simulink model "ejh64a"  (Simulink 3.00)
settings: Solver=ode45  StartTime=0.0  StopTime=15.0  RelTol=1e-3
values from neighbouring files (symbols this model uses):
  K1 = 0.5    [ejh64.m]    (also in ejh65.m)
  K2 = 0.8    [ejh64.m]    (also in ejh65.m)
  x_camino = 0:0.01:10    [ejh64.m]    (also in ejh65.m)
  y_camino = x_camino.^2    [ejh64.m]    (also in ejh65.m)
libraries: simulink_extras x3, dspstat x1
settings Model: OptimizeBlockIOStorage=off  LastModifiedBy=Administrador

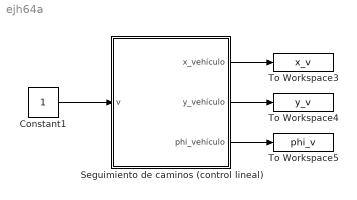
== system ejh64a ==
  Constant1 : Constant  Value=1
  Seguimiento de caminos (control lineal) : Subsystem  mask(Seguimiento de caminos empleando una ley de control lineal){x_inicial=0, y_inicial=0, phi_inicial=0, K1=K1, K2=K2, x_camino=x_camino, y_camino=y_camino}
      mask prompts: x_inicial "Coordenada x inicial del móvil:"; y_inicial "Coordenada y inicial del móvil:"; phi_inicial "Valor inicial de la orientación del móvil:"; K1 "Parámetro K1:"; K2 "Parámetro K2:"; x_camino "Vector con las coordenadas x del camino:"; y_camino "Vector con las coordenadas y del camino:"
      mask help:
      | Este bloque permite simular una estrategia de control lineal para el seguimiento de caminos.
      | A la entrada se dispone de la velocidad del vehículo en cada instante y mediante los parámetros es posible introducir las coordenadas (x,y) del camino. A la salida se obtienen las coordenadas y orientación del vehículo en cada instante.
      mask init:
      | der_x = diff(x_camino);
      | der_y = diff(y_camino);
  To Workspace3 : ToWorkspace  VariableName=x_v  SampleTime=-1  SaveFormat=Matrix
  To Workspace4 : ToWorkspace  VariableName=y_v  SampleTime=-1  SaveFormat=Matrix
  To Workspace5 : ToWorkspace  VariableName=phi_v  SampleTime=-1  SaveFormat=Matrix
  wires:
  Constant1/1 -> Seguimiento de caminos (control lineal)/1(v)
  Seguimiento de caminos (control lineal)/1(x_vehículo) -> To Workspace3/1
  Seguimiento de caminos (control lineal)/3(phi_vehículo) -> To Workspace5/1
  Seguimiento de caminos (control lineal)/2(y_vehículo) -> To Workspace4/1

== system ejh64a/Seguimiento de caminos (control lineal) ==
  v : Inport  Port=1  PortWidth=-1  SampleTime=-1  DataType=auto
      settings: SignalType=auto
  Configuracion síncrona : Subsystem
  Constant : Constant  Value=x_camino
  Constant1 : Constant  Value=y_camino
  Controlador lineal : Subsystem  Orientation=left
  Convertidor : Subsystem  Orientation=left
      mask Description: Este bloque permite transformar la salida del controlador a una señal que será adecuada al vehículo que se desea controlar
  Cálculo de parámetros : Subsystem
  x_vehículo : Outport  Port=1
  y_vehículo : Outport  Port=2
  phi_vehículo : Outport  Port=3
  wires:
  Configuracion síncrona/3(phi_vehículo) -> phi_vehículo/1, Cálculo de parámetros/5(phi_vehiculo)
  Cálculo de parámetros/3(R_c) -> Convertidor/1(R_c)
  v/1 -> Convertidor/3(v), Controlador lineal/2(v), Configuracion síncrona/1(v)
  Configuracion síncrona/2(y_vehículo) -> y_vehículo/1, Cálculo de parámetros/4(y_vehiculo)
  Configuracion síncrona/1(x_vehículo) -> x_vehículo/1, Cálculo de parámetros/3(x_vehiculo)
  Convertidor/1(w) -> Configuracion síncrona/2(w)
  Cálculo de parámetros/1(epsilon) -> Controlador lineal/3(epsilon)
  Controlador lineal/1(u_cont) -> Convertidor/4(u_cont)
  Cálculo de parámetros/2(fi_gorro) -> Convertidor/2(fi_gorro), Controlador lineal/1(fi_gorro)
  Constant1/1 -> Cálculo de parámetros/2(y_camino)
  Constant/1 -> Cálculo de parámetros/1(x_camino)

== system ejh64a/Seguimiento de caminos (control lineal)/Configuracion síncrona ==
  v : Inport  Port=1  PortWidth=-1  SampleTime=-1  DataType=auto
      settings: SignalType=auto
  w : Inport  Port=2  PortWidth=-1  SampleTime=-1  DataType=auto
      settings: SignalType=auto
  Fcn : Fcn  Expr=-sin(u)
  Fcn1 : Fcn  Expr=cos(u)
  Integrator : Integrator  ExternalReset=none  InitialConditionSource=internal  InitialCondition=phi_inicial  LimitOutput=off  UpperSaturationLimit=inf  LowerSaturationLimit=-inf  ShowSaturationPort=off  ShowStatePort=off  AbsoluteTolerance=auto
  Integrator1 : Integrator  ExternalReset=none  InitialConditionSource=internal  InitialCondition=x_inicial  LimitOutput=off  UpperSaturationLimit=inf  LowerSaturationLimit=-inf  ShowSaturationPort=off  ShowStatePort=off  AbsoluteTolerance=auto
  Integrator2 : Integrator  ExternalReset=none  InitialConditionSource=internal  InitialCondition=y_inicial  LimitOutput=off  UpperSaturationLimit=inf  LowerSaturationLimit=-inf  ShowSaturationPort=off  ShowStatePort=off  AbsoluteTolerance=auto
  Product : Product  Inputs=2  SaturateOnIntegerOverflow=on
  Product1 : Product  Inputs=2  SaturateOnIntegerOverflow=on
  x_vehículo : Outport  Port=1
  y_vehículo : Outport  Port=2
  phi_vehículo : Outport  Port=3
  wires:
  Fcn1/1 -> Product1/2
  w/1 -> Integrator/1
  v/1 -> Product1/1, Product/1
  Integrator2/1 -> y_vehículo/1
  Integrator1/1 -> x_vehículo/1
  Integrator/1 -> phi_vehículo/1, Fcn1/1, Fcn/1
  Fcn/1 -> Product/2
  Product/1 -> Integrator1/1
  Product1/1 -> Integrator2/1

== system ejh64a/Seguimiento de caminos (control lineal)/Controlador lineal ==
  fi_gorro : Inport  Port=1  PortWidth=-1  SampleTime=-1  DataType=auto
      settings: SignalType=auto
  v : Inport  Port=2  PortWidth=-1  SampleTime=-1  DataType=auto
      settings: SignalType=auto
  epsilon : Inport  Port=3  PortWidth=-1  SampleTime=-1  DataType=auto
      settings: SignalType=auto
  Abs : Abs
  Gain : Gain  Gain=K1  SaturateOnIntegerOverflow=on
  Gain1 : Gain  Gain=K2  SaturateOnIntegerOverflow=on
  Product : Product  Inputs=2  SaturateOnIntegerOverflow=on
  Product1 : Product  Inputs=2  SaturateOnIntegerOverflow=on
  Sum : Sum  Inputs=--  SaturateOnIntegerOverflow=on
  u_cont : Outport  Port=1  InitialOutput=0
  wires:
  Gain/1 -> Product/1
  v/1 -> Product/2, Abs/1
  Gain1/1 -> Product1/1
  Abs/1 -> Product1/2
  Product/1 -> Sum/1
  Product1/1 -> Sum/2
  epsilon/1 -> Gain/1
  Sum/1 -> u_cont/1
  fi_gorro/1 -> Gain1/1

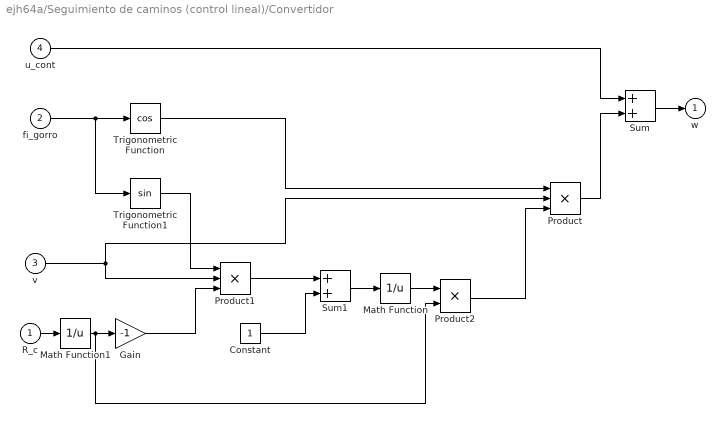
== system ejh64a/Seguimiento de caminos (control lineal)/Convertidor ==
  R_c : Inport  Port=1  PortWidth=-1  SampleTime=-1  DataType=auto
      settings: SignalType=auto
  fi_gorro : Inport  Port=2  PortWidth=-1  SampleTime=-1  DataType=auto
      settings: SignalType=auto
  v : Inport  Port=3  PortWidth=-1  SampleTime=-1  DataType=auto
      settings: SignalType=auto
  u_cont : Inport  Port=4  PortWidth=-1  SampleTime=-1  DataType=auto
      settings: SignalType=auto
  Constant : Constant  Value=1
  Gain : Gain  Gain=-1  SaturateOnIntegerOverflow=on
  Math Function : Math  Operator=reciprocal  OutputSignalType=auto
  Math Function1 : Math  Operator=reciprocal  OutputSignalType=auto
  Product : Product  Inputs=3  SaturateOnIntegerOverflow=on
  Product1 : Product  Inputs=3  SaturateOnIntegerOverflow=on
  Product2 : Product  Inputs=2  SaturateOnIntegerOverflow=on
  Sum : Sum  Inputs=++  SaturateOnIntegerOverflow=on
  Sum1 : Sum  Inputs=++  SaturateOnIntegerOverflow=on
  Trigonometric Function : Trigonometry  Operator=cos  OutputSignalType=auto
  Trigonometric Function1 : Trigonometry  Operator=sin  OutputSignalType=auto
  w : Outport  Port=1  InitialOutput=0
  wires:
  Math Function1/1 -> Gain/1, Product2/2
  R_c/1 -> Math Function1/1
  fi_gorro/1 -> Trigonometric Function/1, Trigonometric Function1/1
  Trigonometric Function1/1 -> Product1/1
  Gain/1 -> Product1/3
  Product1/1 -> Sum1/1
  Constant/1 -> Sum1/2
  Sum1/1 -> Math Function/1
  Trigonometric Function/1 -> Product/1
  v/1 -> Product1/2, Product/2
  Math Function/1 -> Product2/1
  Product/1 -> Sum/2
  u_cont/1 -> Sum/1
  Sum/1 -> w/1
  Product2/1 -> Product/3

== system ejh64a/Seguimiento de caminos (control lineal)/Cálculo de parámetros ==
  x_camino : Inport  Port=1  PortWidth=-1  SampleTime=-1  DataType=auto
      settings: SignalType=auto
  y_camino : Inport  Port=2  PortWidth=-1  SampleTime=-1  DataType=auto
      settings: SignalType=auto
  x_vehiculo : Inport  Port=3  PortWidth=-1  SampleTime=-1  DataType=auto
      settings: SignalType=auto
  y_vehiculo : Inport  Port=4  PortWidth=-1  SampleTime=-1  DataType=auto
      settings: SignalType=auto
  phi_vehiculo : Inport  Port=5  PortWidth=-1  SampleTime=-1  DataType=auto
      settings: SignalType=auto
  Cálculo de phi gorro : Subsystem
  Degrees to Radians : simulink_extras/Transformations/Degrees to Radians
  Subsystem : Subsystem
  epsilon : Outport  Port=1
  fi_gorro : Outport  Port=2
  R_c : Outport  Port=3
  wires:
  x_camino/1 -> Subsystem/1(x_camino)
  y_camino/1 -> Subsystem/2(y_camino)
  y_vehiculo/1 -> Subsystem/4(y_vehiculo)
  x_vehiculo/1 -> Subsystem/3(x_vehiculo)
  Subsystem/3(R_c) -> R_c/1
  phi_vehiculo/1 -> Cálculo de phi gorro/1(fi_vehiculo)
  Degrees to Radians/1 -> fi_gorro/1
  Cálculo de phi gorro/1(fi_go_mo) -> Degrees to Radians/1
  Subsystem/1(distancia) -> epsilon/1
  Subsystem/2(indice) -> Cálculo de phi gorro/2(indice)

== system ejh64a/Seguimiento de caminos (control lineal)/Cálculo de parámetros/Cálculo de phi gorro ==
  fi_vehiculo : Inport  Port=1  PortWidth=-1  SampleTime=-1  DataType=auto
      settings: SignalType=auto
  indice : Inport  Port=2  PortWidth=-1  SampleTime=-1  DataType=auto
      settings: SignalType=auto
  Subsystem : Subsystem
      mask Type: Pasa phi a un ángulo entre -180 y 180
      mask Description: Pasa phi a un ángulo entre -180 y 180
      mask Help: Pasa phi a un ángulo entre -180 y 180
  Subsystem1 : Subsystem
  Subsystem2 : Subsystem
      mask Description: Pasa phi gorro al intervalo -180,180
  suma : Sum  Inputs=+-  SaturateOnIntegerOverflow=on
  fi_go_mo : Outport  Port=1
  wires:
  Subsystem2/1(fi_go_mo) -> fi_go_mo/1
  suma/1 -> Subsystem2/1(fi_gorro)
  Subsystem/1(fi_veh_mod) -> suma/1
  indice/1 -> Subsystem1/1(indice)
  fi_vehiculo/1 -> Subsystem/1(fi_vehiculo)
  Subsystem1/1(fi_camino) -> suma/2

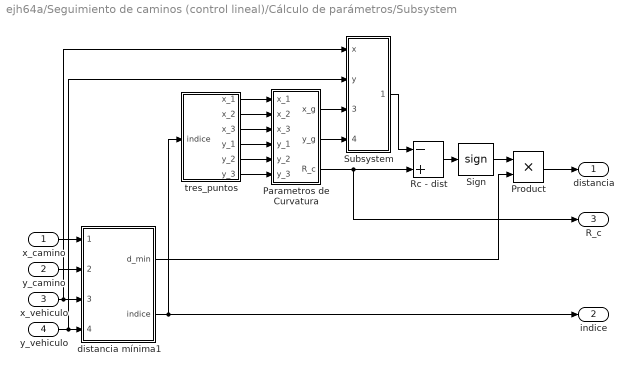
== system ejh64a/Seguimiento de caminos (control lineal)/Cálculo de parámetros/Subsystem ==
  x_camino : Inport  Port=1  PortWidth=-1  SampleTime=-1  DataType=auto
      settings: SignalType=auto
  y_camino : Inport  Port=2  PortWidth=-1  SampleTime=-1  DataType=auto
      settings: SignalType=auto
  x_vehiculo : Inport  Port=3  PortWidth=-1  SampleTime=-1  DataType=auto
      settings: SignalType=auto
  y_vehiculo : Inport  Port=4  PortWidth=-1  SampleTime=-1  DataType=auto
      settings: SignalType=auto
  Parametros de Curvatura : Subsystem
  Product : Product  Inputs=2  SaturateOnIntegerOverflow=on
  Rc - dist : Sum  Inputs=-+  SaturateOnIntegerOverflow=on
  Sign : Signum
  Subsystem : Subsystem
  distancia mínima1 : Subsystem
  tres_puntos : Subsystem
  distancia : Outport  Port=1
  indice : Outport  Port=2
  R_c : Outport  Port=3
  wires:
  distancia mínima1/2(indice) -> tres_puntos/1(indice), indice/1
  Parametros de Curvatura/3(R_c) -> R_c/1, Rc - dist/2
  y_vehiculo/1 -> Subsystem/2(y), distancia mínima1/4(y_vehiculo)
  x_vehiculo/1 -> Subsystem/1(x), distancia mínima1/3(x_vehiculo)
  tres_puntos/4(y_1) -> Parametros de Curvatura/4(y_1)
  tres_puntos/1(x_1) -> Parametros de Curvatura/1(x_1)
  Product/1 -> distancia/1
  y_camino/1 -> distancia mínima1/2(y_camino)
  x_camino/1 -> distancia mínima1/1(x_camino)
  tres_puntos/6(y_3) -> Parametros de Curvatura/6(y_3)
  tres_puntos/5(y_2) -> Parametros de Curvatura/5(y_2)
  tres_puntos/3(x_3) -> Parametros de Curvatura/3(x_3)
  tres_puntos/2(x_2) -> Parametros de Curvatura/2(x_2)
  distancia mínima1/1(d_min) -> Product/2
  Sign/1 -> Product/1
  Parametros de Curvatura/1(x_g) -> Subsystem/3(x_g)
  Parametros de Curvatura/2(y_g) -> Subsystem/4(y_g)
  Subsystem/1(dist) -> Rc - dist/1
  Rc - dist/1 -> Sign/1

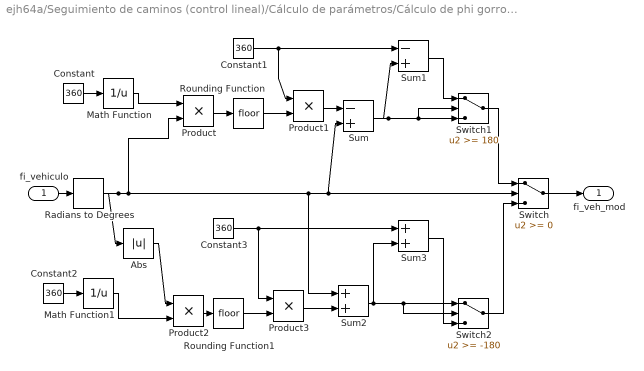
== system ejh64a/Seguimiento de caminos (control lineal)/Cálculo de parámetros/Cálculo de phi gorro/Subsystem ==
  fi_vehiculo : Inport  Port=1  PortWidth=-1  SampleTime=-1  DataType=auto
      settings: SignalType=auto
  Abs : Abs
  Constant{,1..3} (4 alike) : Constant  Value=360
  Math Function : Math  Operator=reciprocal  OutputSignalType=auto
  Math Function1 : Math  Operator=reciprocal  OutputSignalType=auto
  Product{,1..3} (4 alike) : Product  Inputs=2  SaturateOnIntegerOverflow=on
  Radians to Degrees : simulink_extras/Transformations/Radians to Degrees
  Rounding Function : Rounding  Operator=floor
  Rounding Function1 : Rounding  Operator=floor
  Sum : Sum  Inputs=-+  SaturateOnIntegerOverflow=on
  Sum1 : Sum  Inputs=-+  SaturateOnIntegerOverflow=on
  Sum2 : Sum  Inputs=++  SaturateOnIntegerOverflow=on
  Sum3 : Sum  Inputs=++  SaturateOnIntegerOverflow=on
  Switch : Switch  Threshold=0
  Switch1 : Switch  Threshold=180
  Switch2 : Switch  Threshold=-180
  fi_veh_mod : Outport  Port=1
  wires:
  Radians to Degrees/1 -> Abs/1, Sum2/1, Sum/2, Switch/2, Product/2
  fi_vehiculo/1 -> Radians to Degrees/1
  Abs/1 -> Product2/1
  Sum2/1 -> Switch2/2, Switch2/1, Sum3/2
  Sum3/1 -> Switch2/3
  Product2/1 -> Rounding Function1/1
  Math Function1/1 -> Product2/2
  Constant2/1 -> Math Function1/1
  Product3/1 -> Sum2/2
  Rounding Function1/1 -> Product3/2
  Switch2/1 -> Switch/3
  Constant3/1 -> Sum3/1, Product3/1
  Sum1/1 -> Switch1/1
  Sum/1 -> Switch1/2, Switch1/3, Sum1/2
  Constant1/1 -> Sum1/1, Product1/1
  Product1/1 -> Sum/1
  Rounding Function/1 -> Product1/2
  Product/1 -> Rounding Function/1
  Constant/1 -> Math Function/1
  Math Function/1 -> Product/1
  Switch1/1 -> Switch/1
  Switch/1 -> fi_veh_mod/1

== system ejh64a/Seguimiento de caminos (control lineal)/Cálculo de parámetros/Cálculo de phi gorro/Subsystem1 ==
  indice : Inport  Port=1  PortWidth=-1  SampleTime=-1  DataType=auto
      settings: SignalType=auto
  Constant : Constant  Value=90
  Constant1 : Constant  Value=360
  Look-Up Table : Lookup  InputValues=1:length(der_x)  OutputValues=der_x(1:length(der_x))
  Look-Up Table1 : Lookup  InputValues=1:length(der_y)  OutputValues=der_y(1:length(der_y))
  Radians to Degrees : simulink_extras/Transformations/Radians to Degrees
  Sum : Sum  Inputs=+-  SaturateOnIntegerOverflow=on
  Sum1 : Sum  Inputs=++  SaturateOnIntegerOverflow=on
  Switch : Switch  Threshold=-180
  Trigonometric Function : Trigonometry  Operator=atan2  OutputSignalType=auto
  fi_camino : Outport  Port=1
  wires:
  indice/1 -> Look-Up Table/1, Look-Up Table1/1
  Switch/1 -> fi_camino/1
  Sum1/1 -> Switch/3
  Sum/1 -> Switch/2, Sum1/1, Switch/1
  Constant1/1 -> Sum1/2
  Constant/1 -> Sum/2
  Radians to Degrees/1 -> Sum/1
  Trigonometric Function/1 -> Radians to Degrees/1
  Look-Up Table/1 -> Trigonometric Function/2
  Look-Up Table1/1 -> Trigonometric Function/1

== system ejh64a/Seguimiento de caminos (control lineal)/Cálculo de parámetros/Cálculo de phi gorro/Subsystem2 ==
  fi_gorro : Inport  Port=1  PortWidth=-1  SampleTime=-1  DataType=auto
      settings: SignalType=auto
  Constant1 : Constant  Value=360
  Constant2 : Constant  Value=360
  Sum1 : Sum  Inputs=-+  SaturateOnIntegerOverflow=on
  Sum2 : Sum  Inputs=++  SaturateOnIntegerOverflow=on
  Switch : Switch  Threshold=180
  Switch1 : Switch  Threshold=0
  Switch2 : Switch  Threshold=-180
  fi_go_mo : Outport  Port=1
  wires:
  Constant2/1 -> Sum2/2
  fi_gorro/1 -> Sum2/1, Switch2/2, Switch2/1, Switch/2, Switch/3, Switch1/2, Sum1/2
  Sum2/1 -> Switch2/3
  Sum1/1 -> Switch/1
  Constant1/1 -> Sum1/1
  Switch2/1 -> Switch1/3
  Switch/1 -> Switch1/1
  Switch1/1 -> fi_go_mo/1

== system ejh64a/Seguimiento de caminos (control lineal)/Cálculo de parámetros/Subsystem/Parametros de Curvatura ==
  x_1 : Inport  Port=1  PortWidth=-1  SampleTime=-1  DataType=auto
      settings: SignalType=auto
  x_2 : Inport  Port=2  PortWidth=-1  SampleTime=-1  DataType=auto
      settings: SignalType=auto
  x_3 : Inport  Port=3  PortWidth=-1  SampleTime=-1  DataType=auto
      settings: SignalType=auto
  y_1 : Inport  Port=4  PortWidth=-1  SampleTime=-1  DataType=auto
      settings: SignalType=auto
  y_2 : Inport  Port=5  PortWidth=-1  SampleTime=-1  DataType=auto
      settings: SignalType=auto
  y_3 : Inport  Port=6  PortWidth=-1  SampleTime=-1  DataType=auto
      settings: SignalType=auto
  Radio de  Curvatura : Subsystem
  coordenada x c. curvatura : Subsystem
  coordenada y c. curvatura : Subsystem
  x_g : Outport  Port=1  InitialOutput=0
  y_g : Outport  Port=2  InitialOutput=0
  R_c : Outport  Port=3  InitialOutput=0
  wires:
  y_3/1 -> coordenada x c. curvatura/6(y_3), coordenada y c. curvatura/6(y_3)
  y_2/1 -> coordenada y c. curvatura/5(y_2), coordenada x c. curvatura/5(y_2)
  y_1/1 -> Radio de  Curvatura/4(y_1), coordenada x c. curvatura/4(y_1), coordenada y c. curvatura/4(y_1)
  x_3/1 -> coordenada y c. curvatura/3(x_3), coordenada x c. curvatura/3(x_3)
  x_2/1 -> coordenada y c. curvatura/2(x_2), coordenada x c. curvatura/2(x_2)
  x_1/1 -> Radio de  Curvatura/2(x_1), coordenada y c. curvatura/1(x_1), coordenada x c. curvatura/1(x_1)
  coordenada x c. curvatura/1(x_g) -> Radio de  Curvatura/1(x_g), x_g/1
  coordenada y c. curvatura/1(y_g) -> Radio de  Curvatura/3(y_g), y_g/1
  Radio de  Curvatura/1(R_c) -> R_c/1

== system ejh64a/Seguimiento de caminos (control lineal)/Cálculo de parámetros/Subsystem/Subsystem ==
  x : Inport  Port=1  PortWidth=-1  SampleTime=-1  DataType=auto
      settings: SignalType=auto
  y : Inport  Port=2  PortWidth=-1  SampleTime=-1  DataType=auto
      settings: SignalType=auto
  x_g : Inport  Port=3  PortWidth=-1  SampleTime=-1  DataType=auto
      settings: SignalType=auto
  y_g : Inport  Port=4  PortWidth=-1  SampleTime=-1  DataType=auto
      settings: SignalType=auto
  Math Function2 : Math  Operator=sqrt  OutputSignalType=auto
  Math Function3 : Math  Operator=square  OutputSignalType=auto
  Math Function4 : Math  Operator=square  OutputSignalType=auto
  Sum : Sum  Inputs=+-  SaturateOnIntegerOverflow=on
  Sum1 : Sum  Inputs=+-  SaturateOnIntegerOverflow=on
  Sum2 : Sum  Inputs=++  SaturateOnIntegerOverflow=on
  dist : Outport  Port=1  InitialOutput=0
  wires:
  Sum2/1 -> Math Function2/1
  Math Function4/1 -> Sum2/2
  Sum1/1 -> Math Function4/1
  Math Function3/1 -> Sum2/1
  Sum/1 -> Math Function3/1
  y/1 -> Sum1/1
  x_g/1 -> Sum/2
  x/1 -> Sum/1
  y_g/1 -> Sum1/2
  Math Function2/1 -> dist/1

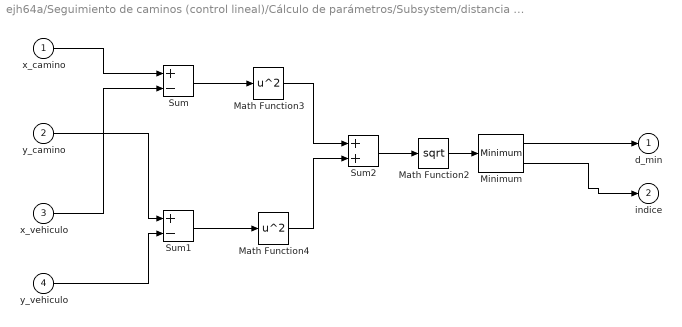
== system ejh64a/Seguimiento de caminos (control lineal)/Cálculo de parámetros/Subsystem/distancia mínima1 ==
  x_camino : Inport  Port=1  PortWidth=-1  SampleTime=-1  DataType=auto
      settings: SignalType=auto
  y_camino : Inport  Port=2  PortWidth=-1  SampleTime=-1  DataType=auto
      settings: SignalType=auto
  x_vehiculo : Inport  Port=3  PortWidth=-1  SampleTime=-1  DataType=auto
      settings: SignalType=auto
  y_vehiculo : Inport  Port=4  PortWidth=-1  SampleTime=-1  DataType=auto
      settings: SignalType=auto
  Math Function2 : Math  Operator=sqrt  OutputSignalType=auto
  Math Function3 : Math  Operator=square  OutputSignalType=auto
  Math Function4 : Math  Operator=square  OutputSignalType=auto
  Minimum : dspstat/Minimum
  Sum : Sum  Inputs=+-  SaturateOnIntegerOverflow=on
  Sum1 : Sum  Inputs=+-  SaturateOnIntegerOverflow=on
  Sum2 : Sum  Inputs=++  SaturateOnIntegerOverflow=on
  d_min : Outport  Port=1  InitialOutput=0
  indice : Outport  Port=2  InitialOutput=0
  wires:
  Minimum/2 -> indice/1
  Minimum/1 -> d_min/1
  Math Function2/1 -> Minimum/1
  Sum2/1 -> Math Function2/1
  Math Function4/1 -> Sum2/2
  Sum1/1 -> Math Function4/1
  Math Function3/1 -> Sum2/1
  Sum/1 -> Math Function3/1
  y_vehiculo/1 -> Sum1/2
  y_camino/1 -> Sum1/1
  x_vehiculo/1 -> Sum/2
  x_camino/1 -> Sum/1

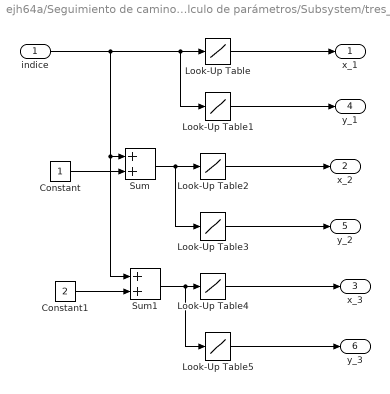
== system ejh64a/Seguimiento de caminos (control lineal)/Cálculo de parámetros/Subsystem/tres_puntos ==
  indice : Inport  Port=1  PortWidth=-1  SampleTime=-1  DataType=auto
      settings: SignalType=auto
  Constant : Constant  Value=1
  Constant1 : Constant  Value=2
  Look-Up Table : Lookup  InputValues=1:length(x_camino)  OutputValues=x_camino(1:length(x_camino))
  Look-Up Table1 : Lookup  InputValues=1:length(y_camino)  OutputValues=y_camino(1:length(y_camino))
  Look-Up Table2 : Lookup  InputValues=1:length(x_camino)  OutputValues=x_camino(1:length(x_camino))
  Look-Up Table3 : Lookup  InputValues=1:length(y_camino)  OutputValues=y_camino(1:length(y_camino))
  Look-Up Table4 : Lookup  InputValues=1:length(x_camino)  OutputValues=x_camino(1:length(x_camino))
  Look-Up Table5 : Lookup  InputValues=1:length(y_camino)  OutputValues=y_camino(1:length(y_camino))
  Sum : Sum  Inputs=++  SaturateOnIntegerOverflow=on
  Sum1 : Sum  Inputs=++  SaturateOnIntegerOverflow=on
  x_1 : Outport  Port=1
  x_2 : Outport  Port=2
  x_3 : Outport  Port=3
  y_1 : Outport  Port=4
  y_2 : Outport  Port=5
  y_3 : Outport  Port=6
  wires:
  Sum1/1 -> Look-Up Table5/1, Look-Up Table4/1
  Look-Up Table4/1 -> x_3/1
  Look-Up Table5/1 -> y_3/1
  Constant1/1 -> Sum1/2
  Look-Up Table1/1 -> y_1/1
  Sum/1 -> Look-Up Table3/1, Look-Up Table2/1
  Look-Up Table3/1 -> y_2/1
  Look-Up Table2/1 -> x_2/1
  Constant/1 -> Sum/2
  indice/1 -> Sum1/1, Sum/1, Look-Up Table1/1, Look-Up Table/1
  Look-Up Table/1 -> x_1/1

== system ejh64a/Seguimiento de caminos (control lineal)/Cálculo de parámetros/Subsystem/Parametros de Curvatura/Radio de  Curvatura ==
  x_g : Inport  Port=1  PortWidth=-1  SampleTime=-1  DataType=auto
      settings: SignalType=auto
  x_1 : Inport  Port=2  PortWidth=-1  SampleTime=-1  DataType=auto
      settings: SignalType=auto
  y_g : Inport  Port=3  PortWidth=-1  SampleTime=-1  DataType=auto
      settings: SignalType=auto
  y_1 : Inport  Port=4  PortWidth=-1  SampleTime=-1  DataType=auto
      settings: SignalType=auto
  Math Function : Math  Operator=square  OutputSignalType=auto
  Math Function1 : Math  Operator=sqrt  OutputSignalType=auto
  Math Function2 : Math  Operator=square  OutputSignalType=auto
  Sum : Sum  Inputs=+-  SaturateOnIntegerOverflow=on
  Sum1 : Sum  Inputs=+-  SaturateOnIntegerOverflow=on
  Sum2 : Sum  Inputs=++  SaturateOnIntegerOverflow=on
  R_c : Outport  Port=1  InitialOutput=0
  wires:
  Math Function1/1 -> R_c/1
  Sum2/1 -> Math Function1/1
  Math Function2/1 -> Sum2/2
  Math Function/1 -> Sum2/1
  Sum1/1 -> Math Function2/1
  Sum/1 -> Math Function/1
  y_g/1 -> Sum1/2
  y_1/1 -> Sum1/1
  x_1/1 -> Sum/1
  x_g/1 -> Sum/2

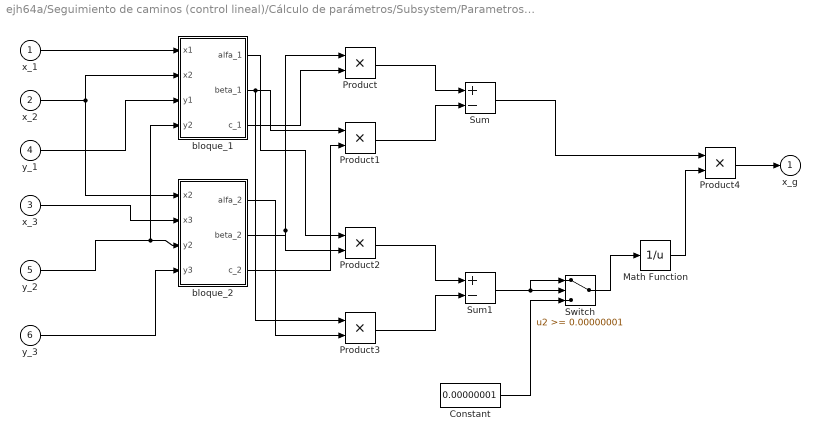
== system ejh64a/Seguimiento de caminos (control lineal)/Cálculo de parámetros/Subsystem/Parametros de Curvatura/coordenada x c. curvatura ==
  x_1 : Inport  Port=1  PortWidth=-1  SampleTime=-1  DataType=auto
      settings: SignalType=auto
  x_2 : Inport  Port=2  PortWidth=-1  SampleTime=-1  DataType=auto
      settings: SignalType=auto
  x_3 : Inport  Port=3  PortWidth=-1  SampleTime=-1  DataType=auto
      settings: SignalType=auto
  y_1 : Inport  Port=4  PortWidth=-1  SampleTime=-1  DataType=auto
      settings: SignalType=auto
  y_2 : Inport  Port=5  PortWidth=-1  SampleTime=-1  DataType=auto
      settings: SignalType=auto
  y_3 : Inport  Port=6  PortWidth=-1  SampleTime=-1  DataType=auto
      settings: SignalType=auto
  Constant : Constant  Value=0.00000001
  Math Function : Math  Operator=reciprocal  OutputSignalType=auto
  Product{,1..4} (5 alike) : Product  Inputs=2  SaturateOnIntegerOverflow=on
  Sum : Sum  Inputs=+-  SaturateOnIntegerOverflow=on
  Sum1 : Sum  Inputs=+-  SaturateOnIntegerOverflow=on
  Switch : Switch  Threshold=0.00000001
  bloque_1 : Subsystem
  bloque_2 : Subsystem
  x_g : Outport  Port=1  InitialOutput=0
  wires:
  Switch/1 -> Math Function/1
  Constant/1 -> Switch/3
  Sum1/1 -> Switch/1, Switch/2
  Product4/1 -> x_g/1
  Product/1 -> Sum/1
  Product1/1 -> Sum/2
  Product2/1 -> Sum1/1
  Product3/1 -> Sum1/2
  Math Function/1 -> Product4/2
  bloque_1/3(c_1) -> Product/2
  bloque_2/3(c_2) -> Product1/2
  bloque_2/2(beta_2) -> Product/1, Product2/2
  bloque_1/1(alfa_1) -> Product2/1
  bloque_1/2(beta_1) -> Product1/1, Product3/1
  bloque_2/1(alfa_2) -> Product3/2
  x_1/1 -> bloque_1/1(x1)
  x_2/1 -> bloque_1/2(x2), bloque_2/1(x2)
  y_1/1 -> bloque_1/3(y1)
  x_3/1 -> bloque_2/2(x3)
  y_2/1 -> bloque_2/3(y2), bloque_1/4(y2)
  y_3/1 -> bloque_2/4(y3)
  Sum/1 -> Product4/1

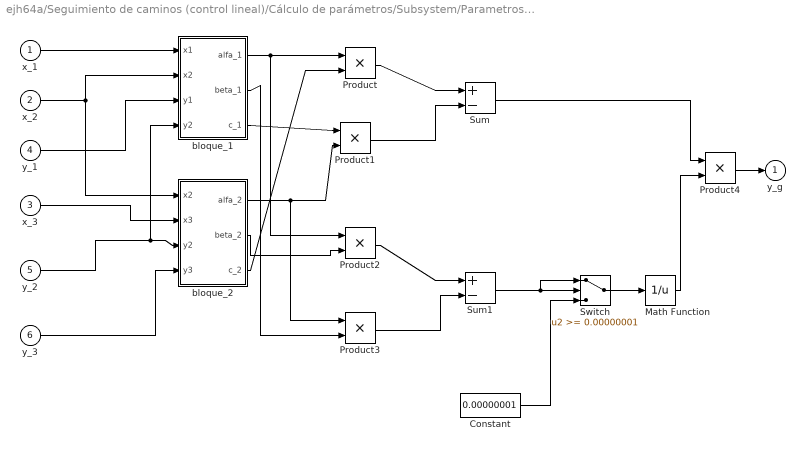
== system ejh64a/Seguimiento de caminos (control lineal)/Cálculo de parámetros/Subsystem/Parametros de Curvatura/coordenada y c. curvatura ==
  x_1 : Inport  Port=1  PortWidth=-1  SampleTime=-1  DataType=auto
      settings: SignalType=auto
  x_2 : Inport  Port=2  PortWidth=-1  SampleTime=-1  DataType=auto
      settings: SignalType=auto
  x_3 : Inport  Port=3  PortWidth=-1  SampleTime=-1  DataType=auto
      settings: SignalType=auto
  y_1 : Inport  Port=4  PortWidth=-1  SampleTime=-1  DataType=auto
      settings: SignalType=auto
  y_2 : Inport  Port=5  PortWidth=-1  SampleTime=-1  DataType=auto
      settings: SignalType=auto
  y_3 : Inport  Port=6  PortWidth=-1  SampleTime=-1  DataType=auto
      settings: SignalType=auto
  Constant : Constant  Value=0.00000001
  Math Function : Math  Operator=reciprocal  OutputSignalType=auto
  Product{,1..4} (5 alike) : Product  Inputs=2  SaturateOnIntegerOverflow=on
  Sum : Sum  Inputs=+-  SaturateOnIntegerOverflow=on
  Sum1 : Sum  Inputs=+-  SaturateOnIntegerOverflow=on
  Switch : Switch  Threshold=0.00000001
  bloque_1 : Subsystem
  bloque_2 : Subsystem
  y_g : Outport  Port=1  InitialOutput=0
  wires:
  Constant/1 -> Switch/3
  Sum1/1 -> Switch/1, Switch/2
  Switch/1 -> Math Function/1
  Math Function/1 -> Product4/2
  Product4/1 -> y_g/1
  bloque_2/3(c_2) -> Product/2
  bloque_1/3(c_1) -> Product1/1
  bloque_1/1(alfa_1) -> Product/1, Product2/1
  bloque_2/2(beta_2) -> Product2/2
  bloque_1/2(beta_1) -> Product3/2
  bloque_2/1(alfa_2) -> Product1/2, Product3/1
  Product/1 -> Sum/1
  Product1/1 -> Sum/2
  Product2/1 -> Sum1/1
  Product3/1 -> Sum1/2
  x_1/1 -> bloque_1/1(x1)
  x_2/1 -> bloque_1/2(x2), bloque_2/1(x2)
  y_1/1 -> bloque_1/3(y1)
  x_3/1 -> bloque_2/2(x3)
  y_2/1 -> bloque_2/3(y2), bloque_1/4(y2)
  y_3/1 -> bloque_2/4(y3)
  Sum/1 -> Product4/1

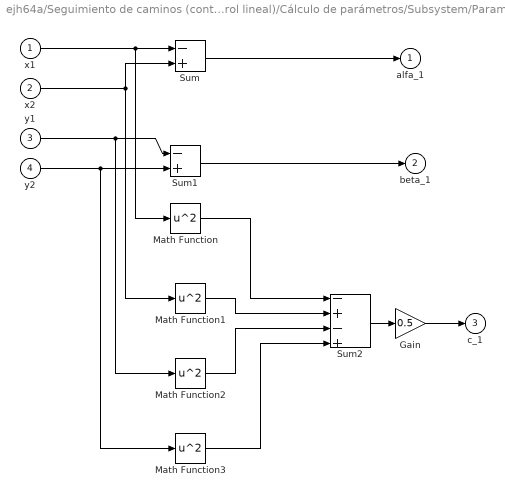
== system ejh64a/Seguimiento de caminos (control lineal)/Cálculo de parámetros/Subsystem/Parametros de Curvatura/coordenada x c. curvatura/bloque_1 ==
  x1 : Inport  Port=1  PortWidth=-1  SampleTime=-1  DataType=auto
      settings: SignalType=auto
  x2 : Inport  Port=2  PortWidth=-1  SampleTime=-1  DataType=auto
      settings: SignalType=auto
  y1 : Inport  Port=3  PortWidth=-1  SampleTime=-1  DataType=auto
      settings: SignalType=auto
  y2 : Inport  Port=4  PortWidth=-1  SampleTime=-1  DataType=auto
      settings: SignalType=auto
  Gain : Gain  Gain=0.5  SaturateOnIntegerOverflow=on
  Math Function{,1..3} (4 alike) : Math  Operator=square  OutputSignalType=auto
  Sum : Sum  Inputs=-+  SaturateOnIntegerOverflow=on
  Sum1 : Sum  Inputs=-+  SaturateOnIntegerOverflow=on
  Sum2 : Sum  Inputs=-+-+  SaturateOnIntegerOverflow=on
  alfa_1 : Outport  Port=1  InitialOutput=0
  beta_1 : Outport  Port=2  InitialOutput=0
  c_1 : Outport  Port=3  InitialOutput=0
  wires:
  Sum/1 -> alfa_1/1
  Sum1/1 -> beta_1/1
  x1/1 -> Sum/1, Math Function/1
  x2/1 -> Sum/2, Math Function1/1
  y1/1 -> Sum1/1, Math Function2/1
  y2/1 -> Sum1/2, Math Function3/1
  Math Function/1 -> Sum2/1
  Math Function1/1 -> Sum2/2
  Math Function2/1 -> Sum2/3
  Math Function3/1 -> Sum2/4
  Sum2/1 -> Gain/1
  Gain/1 -> c_1/1

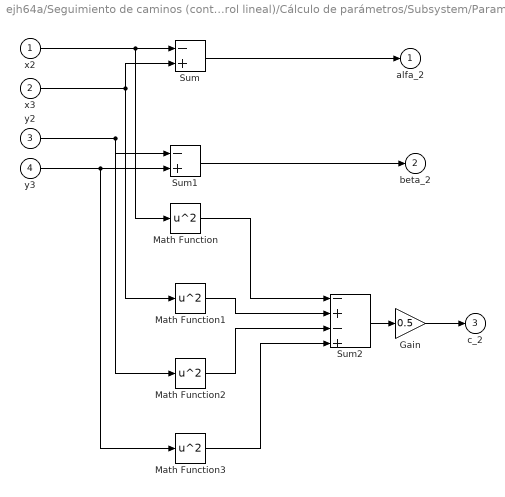
== system ejh64a/Seguimiento de caminos (control lineal)/Cálculo de parámetros/Subsystem/Parametros de Curvatura/coordenada x c. curvatura/bloque_2 ==
  x2 : Inport  Port=1  PortWidth=-1  SampleTime=-1  DataType=auto
      settings: SignalType=auto
  x3 : Inport  Port=2  PortWidth=-1  SampleTime=-1  DataType=auto
      settings: SignalType=auto
  y2 : Inport  Port=3  PortWidth=-1  SampleTime=-1  DataType=auto
      settings: SignalType=auto
  y3 : Inport  Port=4  PortWidth=-1  SampleTime=-1  DataType=auto
      settings: SignalType=auto
  Gain : Gain  Gain=0.5  SaturateOnIntegerOverflow=on
  Math Function{,1..3} (4 alike) : Math  Operator=square  OutputSignalType=auto
  Sum : Sum  Inputs=-+  SaturateOnIntegerOverflow=on
  Sum1 : Sum  Inputs=-+  SaturateOnIntegerOverflow=on
  Sum2 : Sum  Inputs=-+-+  SaturateOnIntegerOverflow=on
  alfa_2 : Outport  Port=1  InitialOutput=0
  beta_2 : Outport  Port=2  InitialOutput=0
  c_2 : Outport  Port=3  InitialOutput=0
  wires:
  Sum/1 -> alfa_2/1
  Sum1/1 -> beta_2/1
  x2/1 -> Sum/1, Math Function/1
  x3/1 -> Sum/2, Math Function1/1
  y2/1 -> Sum1/1, Math Function2/1
  y3/1 -> Sum1/2, Math Function3/1
  Math Function/1 -> Sum2/1
  Math Function1/1 -> Sum2/2
  Math Function2/1 -> Sum2/3
  Math Function3/1 -> Sum2/4
  Sum2/1 -> Gain/1
  Gain/1 -> c_2/1

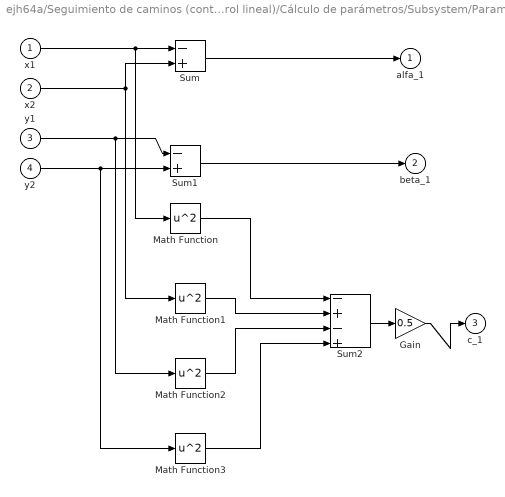
== system ejh64a/Seguimiento de caminos (control lineal)/Cálculo de parámetros/Subsystem/Parametros de Curvatura/coordenada y c. curvatura/bloque_1 ==
  x1 : Inport  Port=1  PortWidth=-1  SampleTime=-1  DataType=auto
      settings: SignalType=auto
  x2 : Inport  Port=2  PortWidth=-1  SampleTime=-1  DataType=auto
      settings: SignalType=auto
  y1 : Inport  Port=3  PortWidth=-1  SampleTime=-1  DataType=auto
      settings: SignalType=auto
  y2 : Inport  Port=4  PortWidth=-1  SampleTime=-1  DataType=auto
      settings: SignalType=auto
  Gain : Gain  Gain=0.5  SaturateOnIntegerOverflow=on
  Math Function{,1..3} (4 alike) : Math  Operator=square  OutputSignalType=auto
  Sum : Sum  Inputs=-+  SaturateOnIntegerOverflow=on
  Sum1 : Sum  Inputs=-+  SaturateOnIntegerOverflow=on
  Sum2 : Sum  Inputs=-+-+  SaturateOnIntegerOverflow=on
  alfa_1 : Outport  Port=1  InitialOutput=0
  beta_1 : Outport  Port=2  InitialOutput=0
  c_1 : Outport  Port=3  InitialOutput=0
  wires:
  Sum/1 -> alfa_1/1
  Sum1/1 -> beta_1/1
  x1/1 -> Sum/1, Math Function/1
  x2/1 -> Sum/2, Math Function1/1
  y1/1 -> Sum1/1, Math Function2/1
  y2/1 -> Sum1/2, Math Function3/1
  Math Function/1 -> Sum2/1
  Math Function1/1 -> Sum2/2
  Math Function2/1 -> Sum2/3
  Math Function3/1 -> Sum2/4
  Sum2/1 -> Gain/1
  Gain/1 -> c_1/1

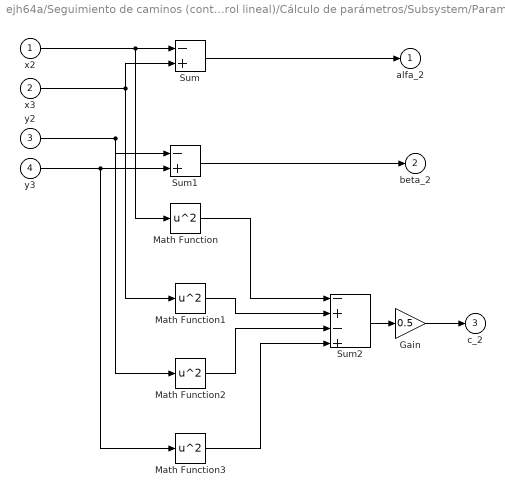
== system ejh64a/Seguimiento de caminos (control lineal)/Cálculo de parámetros/Subsystem/Parametros de Curvatura/coordenada y c. curvatura/bloque_2 ==
  x2 : Inport  Port=1  PortWidth=-1  SampleTime=-1  DataType=auto
      settings: SignalType=auto
  x3 : Inport  Port=2  PortWidth=-1  SampleTime=-1  DataType=auto
      settings: SignalType=auto
  y2 : Inport  Port=3  PortWidth=-1  SampleTime=-1  DataType=auto
      settings: SignalType=auto
  y3 : Inport  Port=4  PortWidth=-1  SampleTime=-1  DataType=auto
      settings: SignalType=auto
  Gain : Gain  Gain=0.5  SaturateOnIntegerOverflow=on
  Math Function{,1..3} (4 alike) : Math  Operator=square  OutputSignalType=auto
  Sum : Sum  Inputs=-+  SaturateOnIntegerOverflow=on
  Sum1 : Sum  Inputs=-+  SaturateOnIntegerOverflow=on
  Sum2 : Sum  Inputs=-+-+  SaturateOnIntegerOverflow=on
  alfa_2 : Outport  Port=1  InitialOutput=0
  beta_2 : Outport  Port=2  InitialOutput=0
  c_2 : Outport  Port=3  InitialOutput=0
  wires:
  Sum/1 -> alfa_2/1
  Sum1/1 -> beta_2/1
  x2/1 -> Sum/1, Math Function/1
  x3/1 -> Sum/2, Math Function1/1
  y2/1 -> Sum1/1, Math Function2/1
  y3/1 -> Sum1/2, Math Function3/1
  Math Function/1 -> Sum2/1
  Math Function1/1 -> Sum2/2
  Math Function2/1 -> Sum2/3
  Math Function3/1 -> Sum2/4
  Sum2/1 -> Gain/1
  Gain/1 -> c_2/1
